simulink model "plead"  (R2021a)
settings: Solver=VariableStepAuto  StartTime=0.0  StopTime=10.0  RelTol=1e-3
settings Model: Creator=Ajay M  LastModifiedBy=Ajay M

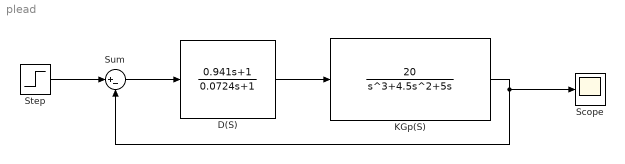
== system plead ==
  D(S) : TransferFcn  Numerator=[0.941 1]  Denominator=[0.0724 1]
  KGp(S) : TransferFcn  Numerator=[20]  Denominator=[1 4.5 5 0]
  Scope : Scope
  Step : Step  SampleTime=0
  Sum : Sum  Inputs=|+-
  wires:
  D(S)/1 -> KGp(S)/1
  Sum/1 -> D(S)/1
  Step/1 -> Sum/1
  KGp(S)/1 -> Scope/1, Sum/2
